simulink model "pmsm_dis_modified"  (R2019a)
settings: Solver=ode3  StartTime=0.0  StopTime=30  FixedStep=Ts  RelTol=1e-3  EnableMultiTasking=on
InitFcn:
  | Ts=1e-3;
settings Model: Creator=srikanth  LastModifiedBy=gfretti
settings DataIOCC: LimitDataPoints=on  SaveFormat=Array  ReturnWorkspaceOutputs=off
settings OptimizationCC: ExpressionDepthLimit=2147483647  LifeSpan=inf
settings DebuggingCC: UnderspecifiedInitializationDetection=Classic  MergeDetectMultiDrivingBlocksExec=none  SolverPrmCheckMsg=warning  FcnCallInpInsideContextMsg=warning  StateNameClashWarn=warning  SFUnexpectedBacktrackingDiag=warning  SFNoUnconditionalDefaultTransitionDiag=warning  SFExecutionAtInitializationDiag=none  ArithmeticOperatorsInVariantConditions=warning
settings HardwareCC: ProdBitPerPointer=32  ProdBitPerSizeT=32  ProdBitPerPtrDiffT=32  ProdLargestAtomicFloat=None  ProdIntDivRoundTo=Undefined  ProdEndianess=Unspecified  ProdWordSize=32  ProdHWDeviceType=32-bit Generic
settings ModelReferenceCC: PropagateSignalLabelsOutOfModel=off
settings SFSimCC: SimUseLocalCustomCode=off
settings RTWCC: RTWUseLocalCustomCode=off
settings CodeAppCC: StateflowObjectComments=on
settings GRTTargetCC: TargetLangStandard=C89/C90 (ANSI)  CombineOutputUpdateFcns=off  GRTInterface=on
settings ConfigComp: CovMetricSettings=dw  CovHtmlReporting=on  CovSaveCumulativeToWorkspaceVar=on  CovSaveSingleToWorkspaceVar=on  CovExternalEMLEnable=off

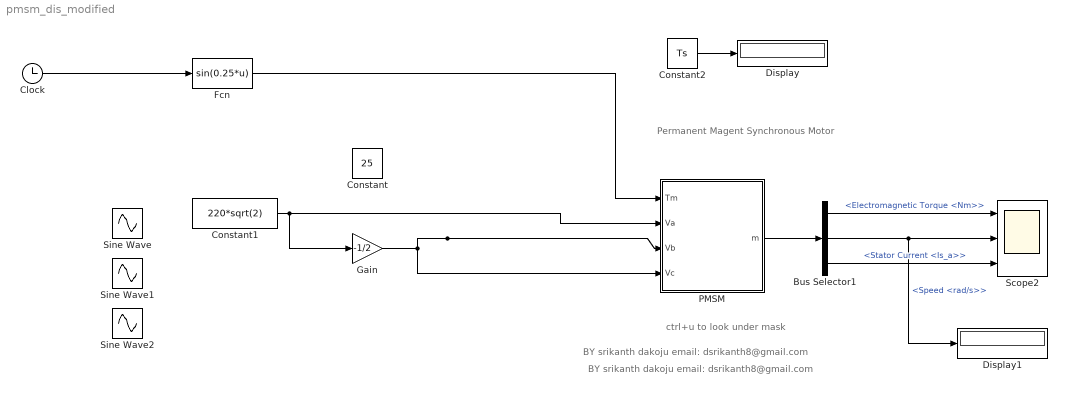
== system pmsm_dis_modified ==
  note: ctrl+u to look under mask
  note: Permanent Magent Synchronous Motor
  note: BY
      | srikanth dakoju
      | email: dsrikanth8@gmail.com
  note: BY
      | srikanth dakoju
      | email: dsrikanth8@gmail.com
  Bus Selector1 : BusSelector  OutputSignals=Electromagnetic Torque <Nm>,Speed <rad/s>,Stator Current <Is_a>
  Clock : Clock
  Constant : Constant  Value=25
  Constant1 : Constant  Value=220*sqrt(2)
  Constant2 : Constant  Value=Ts
  Display : Display
  Display1 : Display
  Fcn : Fcn  Expr=sin(0.25*u)
  Gain : Gain  Gain=-1/2
  PMSM : Subsystem  mask(Permanent Magnet Synchronous Motor :){Rs=0.4578, Ld=0.00333, Lq=0.00334, flux=0.171, J=0.001469, B=0.0003035, p=8}
      mask prompts: Rs "Stator Resistance - Rs [ohm] :"; Ld "Direct axis Inductance - Ld [H]"; Lq "Quadrature axis Inductance - Lq [H] :"; flux "Flux - [Wb]"; J "Rotor Inertia - J [kg-m^2]"; B "Friction Coefficient - B"; p "No: of Poles"
      mask Display: fprintf('PMSM')
  Scope2 : Scope  NumInputPorts=3
  Sine Wave : Sin  Amplitude=220*sqrt(2)  Frequency=2*pi*50  SampleTime=Ts
  Sine Wave1 : Sin  Amplitude=220*sqrt(2)  Frequency=2*pi*50  Phase=-2*pi/3  SampleTime=Ts
  Sine Wave2 : Sin  Amplitude=220*sqrt(2)  Frequency=2*pi*50  Phase=2*pi/3  SampleTime=Ts
  wires:
  PMSM/1(m) -> Bus Selector1/1
  Bus Selector1/1 -> Scope2/1  "<Electromagnetic Torque <Nm>>"
  Bus Selector1/2 -> Scope2/2, Display1/1  "<Speed <rad/s>>"
  Bus Selector1/3 -> Scope2/3  "<Stator Current <Is_a>>"
  Constant1/1 -> PMSM/2(Va), Gain/1
  Gain/1 -> PMSM/4(Vc), PMSM/3(Vb)
  Constant2/1 -> Display/1
  Clock/1 -> Fcn/1
  Fcn/1 -> PMSM/1(Tm)

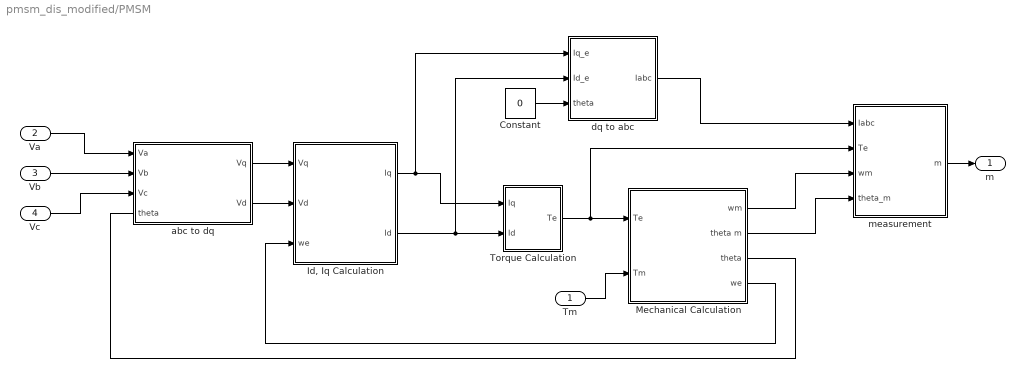
== system pmsm_dis_modified/PMSM ==
  Tm : Inport
  Va : Inport  Port=2
  Vb : Inport  Port=3
  Vc : Inport  Port=4
  Constant : Constant  Value=0
  "Id, Iq Calculation" : Subsystem
  Mechanical Calculation : Subsystem
  Torque Calculation : Subsystem
  abc to dq : Subsystem
  dq to abc : Subsystem
  measurement : Subsystem
  m : Outport
  wires:
  "Id, Iq Calculation"/2(Id) -> Torque Calculation/2(Id), dq to abc/2(Id_e)
  "Id, Iq Calculation"/1(Iq) -> Torque Calculation/1(Iq), dq to abc/1(Iq_e)
  Tm/1 -> Mechanical Calculation/2(Tm)
  abc to dq/1(Vq) -> "Id, Iq Calculation"/1(Vq)
  abc to dq/2(Vd) -> "Id, Iq Calculation"/2(Vd)
  Torque Calculation/1(Te) -> Mechanical Calculation/1(Te), measurement/2(Te)
  Mechanical Calculation/4(we) -> "Id, Iq Calculation"/3(we)
  Mechanical Calculation/3(theta) -> ?
  Va/1 -> abc to dq/1(Va)
  Vb/1 -> abc to dq/2(Vb)
  Vc/1 -> abc to dq/3(Vc)
  dq to abc/1(Iabc) -> measurement/1(Iabc)
  Mechanical Calculation/1(wm) -> measurement/3(wm)
  Mechanical Calculation/2(theta m) -> measurement/4(theta_m)
  measurement/1(m) -> m/1
  Constant/1 -> dq to abc/3(theta)

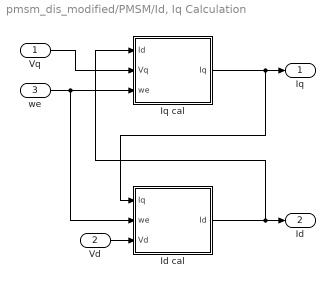
== system pmsm_dis_modified/PMSM/Id, Iq Calculation ==
  Vq : Inport
  Vd : Inport  Port=2
  we : Inport  Port=3
  Id cal : Subsystem
  Iq cal : Subsystem
  Iq : Outport
  Id : Outport  Port=2
  wires:
  Iq cal/1(Iq) -> Id cal/1(Iq), Iq/1
  Id cal/1(Id) -> Iq cal/1(Id), Id/1
  we/1 -> Iq cal/3(we), Id cal/2(we)
  Vq/1 -> Iq cal/2(Vq)
  Vd/1 -> Id cal/3(Vd)

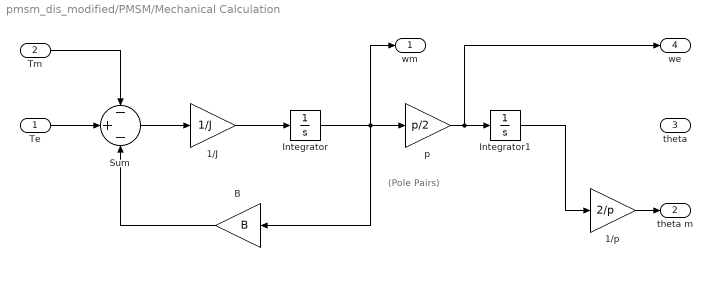
== system pmsm_dis_modified/PMSM/Mechanical Calculation ==
  note: (Pole Pairs)
  Te : Inport
  Tm : Inport  Port=2
  1/J : Gain  Gain=1/J
  1/p : Gain  Gain=2/p
  B : Gain  Gain=B
  Integrator : Integrator
  Integrator1 : Integrator
  Sum : Sum  Inputs=-+-
  p : Gain  Gain=p/2
  wm : Outport
  theta m : Outport  Port=2
  theta : Outport  Port=3
  we : Outport  Port=4
  wires:
  Te/1 -> Sum/2
  Tm/1 -> Sum/1
  Sum/1 -> 1/J/1
  1/J/1 -> Integrator/1
  Integrator/1 -> B/1, p/1, wm/1
  B/1 -> Sum/3
  p/1 -> we/1, Integrator1/1
  Integrator1/1 -> 1/p/1
  1/p/1 -> theta m/1

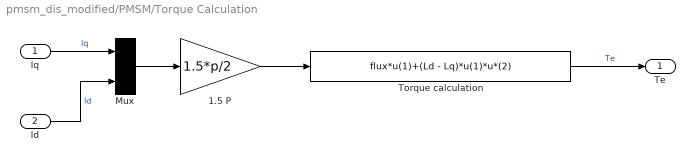
== system pmsm_dis_modified/PMSM/Torque Calculation ==
  Iq : Inport
  Id : Inport  Port=2
  1.5 P : Gain  Gain=1.5*p/2
  Mux : Mux  Inputs=2
      settings: DisplayOption=signals
  Torque calculation : Fcn  Expr=flux*u(1)+(Ld - Lq)*u(1)*u*(2)
  Te : Outport
  wires:
  Torque calculation/1 -> Te/1  "Te"
  Mux/1 -> 1.5 P/1
  Iq/1 -> Mux/1  "Iq"
  Id/1 -> Mux/2  "Id"
  1.5 P/1 -> Torque calculation/1

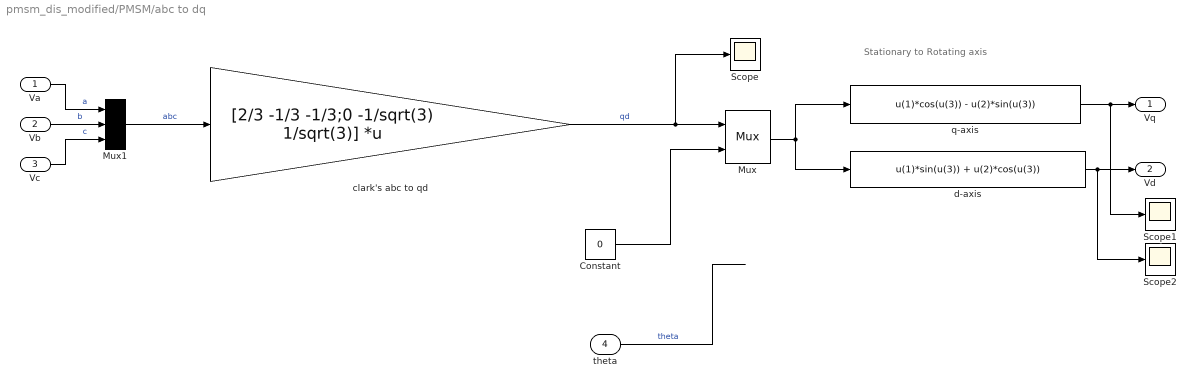
== system pmsm_dis_modified/PMSM/abc to dq ==
  note: Stationary to Rotating axis
  Va : Inport
  Vb : Inport  Port=2
  Vc : Inport  Port=3
  theta : Inport  Port=4
  Constant : Constant  Value=0
  Mux : Mux  Inputs=2
      settings: DisplayOption=signals
  Mux1 : Mux  Inputs=3
      settings: DisplayOption=signals
  Scope : Scope
  Scope1 : Scope
  Scope2 : Scope
  clark's abc to qd : Gain  Gain=[2/3 -1/3 -1/3;0 -1/sqrt(3) 1/sqrt(3)]  Multiplication=Matrix(K*u)
  d-axis : Fcn  Expr=u(1)*sin(u(3)) + u(2)*cos(u(3))
  q-axis : Fcn  Expr=u(1)*cos(u(3)) - u(2)*sin(u(3))
  Vq : Outport
  Vd : Outport  Port=2
  wires:
  Mux/1 -> q-axis/1, d-axis/1
  d-axis/1 -> Scope2/1, Vd/1
  Vc/1 -> Mux1/3  "c"
  Vb/1 -> Mux1/2  "b"
  Va/1 -> Mux1/1  "a"
  q-axis/1 -> Vq/1, Scope1/1
  Mux1/1 -> clark's abc to qd/1  "abc"
  clark's abc to qd/1 -> Scope/1, Mux/1  "qd"
  theta/1 -> ?  "theta"
  Constant/1 -> Mux/2

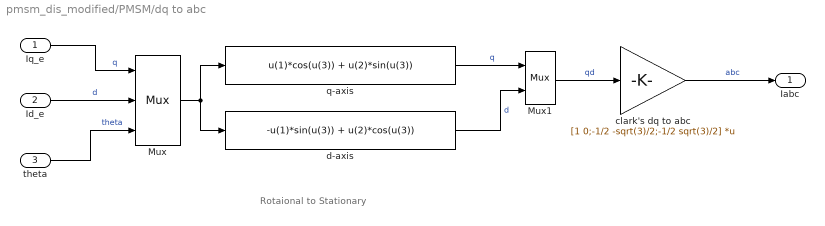
== system pmsm_dis_modified/PMSM/dq to abc ==
  note: Rotaional to Stationary
  Iq_e : Inport
  Id_e : Inport  Port=2
  theta : Inport  Port=3
  Mux : Mux  Inputs=3
      settings: DisplayOption=signals
  Mux1 : Mux  Inputs=2
      settings: DisplayOption=signals
  clark's dq to abc : Gain  Gain=[1 0;-1/2 -sqrt(3)/2;-1/2 sqrt(3)/2]  Multiplication=Matrix(K*u)
  d-axis : Fcn  Expr=-u(1)*sin(u(3)) + u(2)*cos(u(3))
  q-axis : Fcn  Expr=u(1)*cos(u(3)) + u(2)*sin(u(3))
  Iabc : Outport
  wires:
  Mux/1 -> q-axis/1, d-axis/1
  Iq_e/1 -> Mux/1  "q"
  Id_e/1 -> Mux/2  "d"
  theta/1 -> Mux/3  "theta"
  q-axis/1 -> Mux1/1  "q"
  d-axis/1 -> Mux1/2  "d"
  Mux1/1 -> clark's dq to abc/1  "qd"
  clark's dq to abc/1 -> Iabc/1  "abc"

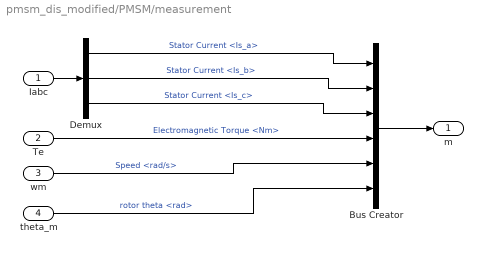
== system pmsm_dis_modified/PMSM/measurement ==
  Iabc : Inport
  Te : Inport  Port=2
  wm : Inport  Port=3
  theta_m : Inport  Port=4
  Bus Creator : BusCreator  Inputs=6
  Demux : Demux  Outputs=3
  m : Outport
  wires:
  Iabc/1 -> Demux/1
  Demux/1 -> Bus Creator/1  "Stator Current <Is_a>"
  Demux/3 -> Bus Creator/3  "Stator Current <Is_c>"
  Te/1 -> Bus Creator/4  "Electromagnetic Torque <Nm>"
  wm/1 -> Bus Creator/5  "Speed <rad/s>"
  theta_m/1 -> Bus Creator/6  "rotor theta <rad>"
  Bus Creator/1 -> m/1
  Demux/2 -> Bus Creator/2  "Stator Current <Is_b>"

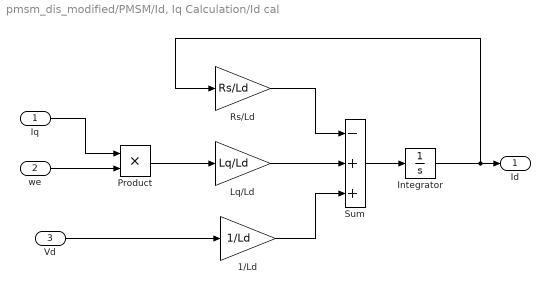
== system pmsm_dis_modified/PMSM/Id, Iq Calculation/Id cal ==
  Iq : Inport
  we : Inport  Port=2
  Vd : Inport  Port=3
  1/Ld : Gain  Gain=1/Ld
  Integrator : Integrator
  Lq/Ld : Gain  Gain=Lq/Ld
  Product : Product  RndMeth=Zero
  Rs/Ld : Gain  Gain=Rs/Ld
  Sum : Sum  Inputs=-++
  Id : Outport
  wires:
  Vd/1 -> 1/Ld/1
  Iq/1 -> Product/1
  we/1 -> Product/2
  Product/1 -> Lq/Ld/1
  Integrator/1 -> Id/1, Rs/Ld/1
  Sum/1 -> Integrator/1
  1/Ld/1 -> Sum/3
  Lq/Ld/1 -> Sum/2
  Rs/Ld/1 -> Sum/1

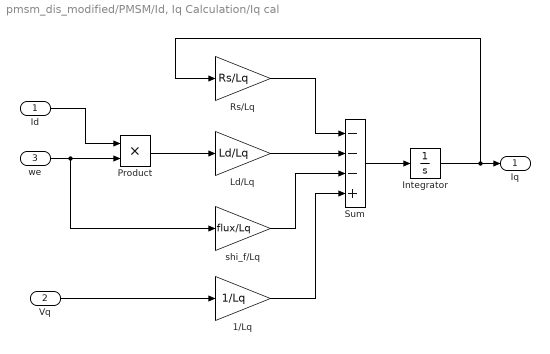
== system pmsm_dis_modified/PMSM/Id, Iq Calculation/Iq cal ==
  Id : Inport
  Vq : Inport  Port=2
  we : Inport  Port=3
  1/Lq : Gain  Gain=1/Lq
  Integrator : Integrator
  Ld/Lq : Gain  Gain=Ld/Lq
  Product : Product  RndMeth=Zero
  Rs/Lq : Gain  Gain=Rs/Lq
  Sum : Sum  Inputs=---+
  shi_f/Lq : Gain  Gain=flux/Lq
  Iq : Outport
  wires:
  Rs/Lq/1 -> Sum/1
  Ld/Lq/1 -> Sum/2
  shi_f/Lq/1 -> Sum/3
  1/Lq/1 -> Sum/4
  Sum/1 -> Integrator/1
  Integrator/1 -> Rs/Lq/1, Iq/1
  Product/1 -> Ld/Lq/1
  we/1 -> Product/2, shi_f/Lq/1
  Id/1 -> Product/1
  Vq/1 -> 1/Lq/1
